simulink model "exampleMinRunTime2"  (Simulink 7.6)
settings: Solver=ode45  StartTime=0.0  StopTime=30  RelTol=1e-3
undefined symbols (not defined in the file): minruntime
libraries: simulink x2
settings Model: Creator=drhf  LastModifiedBy=drhf

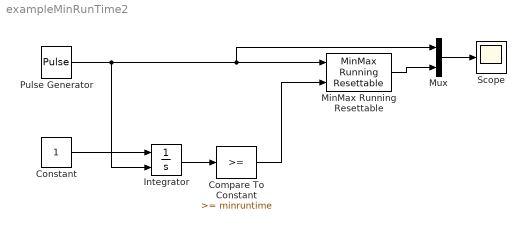
== system exampleMinRunTime2 ==
  Compare To Constant : simulink/Logic and Bit Operations/Compare To Constant  SystemSampleTime=-1  relop=>=  const=minruntime  LogicOutDataTypeMode=uint8
  Constant : Constant
  Integrator : Integrator  ExternalReset=rising
  MinMax Running Resettable : simulink/Math Operations/MinMax Running Resettable  SystemSampleTime=-1  Function=max  vinit=0.0
  Mux : Mux  Inputs=2
  Pulse Generator : DiscretePulseGenerator  PulseType=Time based  Period=10  PulseWidth=5
  Scope : Scope
  wires:
  Constant/1 -> Integrator/1
  Pulse Generator/1 -> Integrator/2, MinMax Running Resettable/1, Mux/1
  Integrator/1 -> Compare To Constant/1
  Compare To Constant/1 -> MinMax Running Resettable/2
  Mux/1 -> Scope/1
  MinMax Running Resettable/1 -> Mux/2
